simulink model "gm_motor_dtf"  (R2021b)
settings: Solver=FixedStepDiscrete  StartTime=0.0  StopTime=500  RelTol=1e-3
undefined symbols (not defined in the file or in its folder): DiscIntNeverNeededParam
Description:
  | Symmetric FIR Filter
  | This example shows how to use HDL Coder(TM) to check, generate,
  | and verify HDL for a fixed-point symmetric FIR filter.
settings Model: Creator=The MathWorks, Inc.  LastModifiedBy=Marco Milanesi
settings SolverCC: AlgebraicLoopSolver=TrustRegion
settings DataIOCC: LimitDataPoints=on  SaveFormat=Array  SaveOutput=off  SignalLogging=off  SaveTime=off  ReturnWorkspaceOutputs=off  SignalLoggingName=logsOut
settings OptimizationCC: BlockReduction=off  BooleanDataType=off  ConditionallyExecuteInputs=off  DefaultParameterBehavior=Inlined  InheritOutputTypeSmallerThanSingle=on  InlineInvariantSignals=on  ExpressionDepthLimit=2147483647  InitFltsAndDblsToZero=on  LifeSpan=inf  BufferReusableBoundary=off
settings DebuggingCC: AlgebraicLoopMsg=error  SaveWithParameterizedLinksMsg=none  UnderspecifiedInitializationDetection=Classic  MergeDetectMultiDrivingBlocksExec=none  CheckExecutionContextPreStartOutputMsg=on  SignalResolutionControl=TryResolveAllWithWarning  InheritedTsInSrcMsg=none  MultiTaskDSMMsg=warning  MultiTaskCondExecSysMsg=none  SingleTaskRateTransMsg=error  IntegerOverflowMsg=none  ParameterPrecisionLossMsg=none  FcnCallInpInsideContextMsg=warning  BusObjectLabelMismatch=none  StateNameClashWarn=warning  SFUnexpectedBacktrackingDiag=warning  SFNoUnconditionalDefaultTransitionDiag=warning  SFExecutionAtInitializationDiag=none  SFMachineParentedDataDiag=warning  IntegerSaturationMsg=none  ArithmeticOperatorsInVariantConditions=warning
settings HardwareCC: ProdBitPerPointer=32  ProdBitPerSizeT=32  ProdBitPerPtrDiffT=32  ProdLargestAtomicFloat=None  ProdIntDivRoundTo=Undefined  ProdEndianess=Unspecified  ProdWordSize=32  ProdHWDeviceType=ASIC/FPGA  TargetUnknown=on  ProdEqTarget=off
settings ModelReferenceCC: PropagateSignalLabelsOutOfModel=off
settings SFSimCC: SimUseLocalCustomCode=off  CustomCodeUndefinedFunction=UseInterfaceOnly
settings RTWCC: RTWUseLocalCustomCode=off
settings CodeAppCC: StateflowObjectComments=on
settings GRTTargetCC: TargetFcnLib=ansi_tfl_tmw.mat  TargetLangStandard=C89/C90 (ANSI)  CombineOutputUpdateFcns=off  GRTInterface=on
settings ConfigComp: CovMetricSettings=dw  CovSaveCumulativeToWorkspaceVar=on  CovSaveSingleToWorkspaceVar=on  CovExternalEMLEnable=off

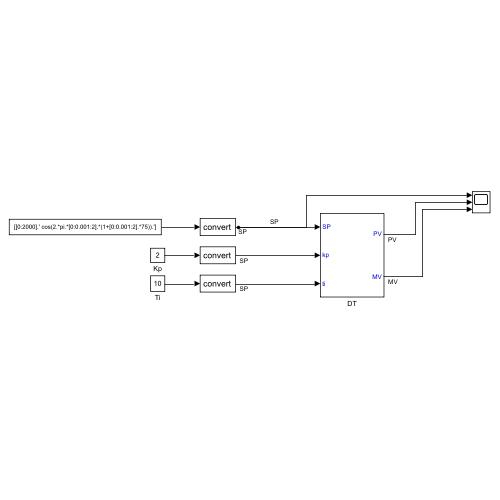
[thumbnail: Simulink's stored preview of the top-level diagram]
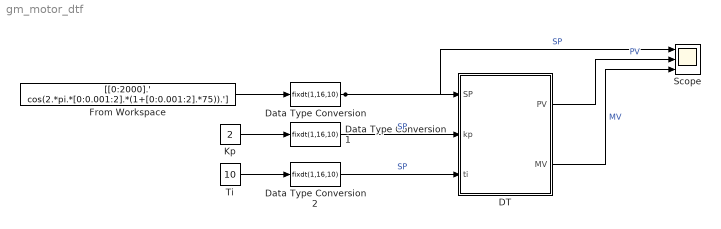
== system gm_motor_dtf ==
  DT : Subsystem
  Data Type Conversion : DataTypeConversion  OutDataTypeStr=fixdt(1,16,10)
  Data Type Conversion1 : DataTypeConversion  OutDataTypeStr=fixdt(1,16,10)
  Data Type Conversion2 : DataTypeConversion  OutDataTypeStr=fixdt(1,16,10)
  From Workspace : FromWorkspace  VariableName=[[0:2000].' cos(2.*pi.*[0:0.001:2].*(1+[0:0.001:2].*75)).']  SampleTime=1  OutputAfterFinalValue=Setting to zero
  Kp : Constant  Value=2
  Scope : Scope  NumInputPorts=3
  Ti : Constant  Value=10
  wires:
  Ti/1 -> Data Type Conversion2/1
  Data Type Conversion2/1 -> DT/3(ti)  "SP"
  Data Type Conversion1/1 -> DT/2(kp)  "SP"
  Kp/1 -> Data Type Conversion1/1
  DT/2(MV) -> Scope/3  "MV"
  Data Type Conversion/1 -> DT/1(SP), Scope/1  "SP"
  From Workspace/1 -> Data Type Conversion/1
  DT/1(PV) -> Scope/2  "PV"

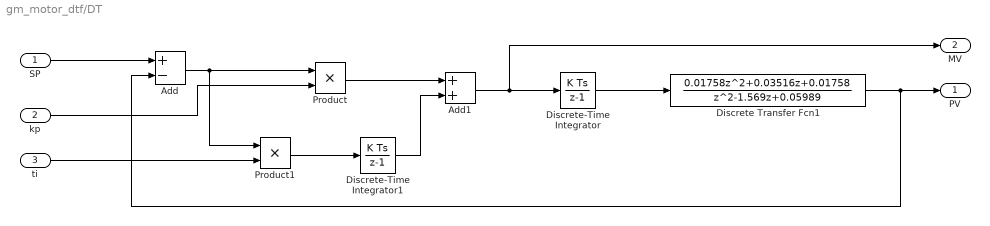
== system gm_motor_dtf/DT ==
  SP : Inport
  kp : Inport  Port=2
  ti : Inport  Port=3
  Add : Sum  Inputs=+-  AccumDataTypeStr=fixdt(1,16,10)  OutDataTypeStr=fixdt(1,16,10)
  Add1 : Sum  AccumDataTypeStr=fixdt(1,16,10)  OutDataTypeStr=fixdt(1,16,10)
  Discrete Transfer Fcn1 : DiscreteTransferFcn  Numerator=[0.01758, 0.03516, 0.01758]  Denominator=[1,-1.569, 0.05989]  NumCoefDataTypeStr=fixdt(1,16,10)  DenCoefDataTypeStr=fixdt(1,16,10)  NumProductDataTypeStr=fixdt(1,16,10)  DenProductDataTypeStr=fixdt(1,16,10)  NumAccumDataTypeStr=fixdt(1,16,10)  DenAccumDataTypeStr=fixdt(1,16,10)  OutDataTypeStr=fixdt(1,16,10)
  Discrete-Time Integrator : DiscreteIntegrator  SampleTime=-1  OutDataTypeStr=fixdt(1,16,10)  ICPrevOutput=DiscIntNeverNeededParam  ICPrevScaledInput=DiscIntNeverNeededParam
  Discrete-Time Integrator1 : DiscreteIntegrator  SampleTime=-1  OutDataTypeStr=fixdt(1,16,10)  ICPrevOutput=DiscIntNeverNeededParam  ICPrevScaledInput=DiscIntNeverNeededParam
  Product : Product  OutDataTypeStr=fixdt(1,16,10)
  Product1 : Product  OutDataTypeStr=fixdt(1,16,10)
  PV : Outport  VectorParamsAs1DForOutWhenUnconnected=off
  MV : Outport  Port=2  VectorParamsAs1DForOutWhenUnconnected=off
  wires:
  Discrete-Time Integrator/1 -> Discrete Transfer Fcn1/1
  Add1/1 -> Discrete-Time Integrator/1, MV/1
  Discrete-Time Integrator1/1 -> Add1/2
  Product1/1 -> Discrete-Time Integrator1/1
  ti/1 -> Product1/2
  Product/1 -> Add1/1
  kp/1 -> Product/2
  Add/1 -> Product1/1, Product/1
  Discrete Transfer Fcn1/1 -> PV/1, Add/2
  SP/1 -> Add/1
